simulink model "tractor_trailer_kinematics"  (R2024b)
settings: Solver=FixedStepAuto  StartTime=0.0  StopTime=10.0  FixedStep=0.01  RelTol=1e-3
values from neighbouring files (symbols this model uses):
  init_yaw = data.YawRad(1)    [initialize.m]
undefined symbols (not defined in the file or in its folder): param
settings Model: Creator=matve  LastModifiedBy=matve
settings RTWCC: GPUComputeCapability=3.5

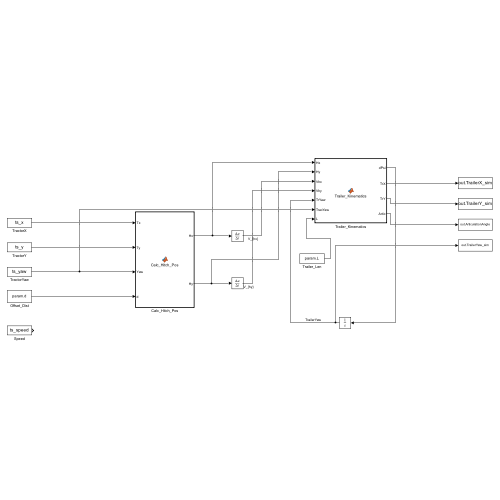
[thumbnail: Simulink's stored preview of the top-level diagram]
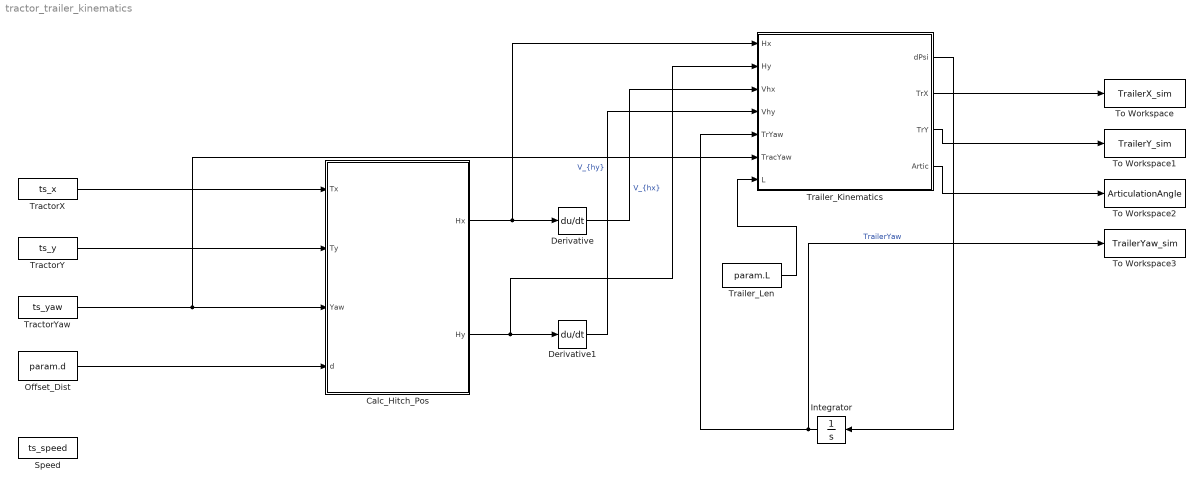
== system tractor_trailer_kinematics ==
  Calc_Hitch_Pos : MATLAB Function  TreatAsAtomicUnit=on
  Derivative : Derivative
  Derivative1 : Derivative
  Integrator : Integrator  InitialCondition=init_yaw
  Offset_Dist : Constant  Value=param.d
  Speed : FromWorkspace  VariableName=ts_speed  OutputAfterFinalValue=Holding final value
  To Workspace : ToWorkspace  VariableName=TrailerX_sim  SaveFormat=Timeseries  SampleTime=-1
  To Workspace1 : ToWorkspace  VariableName=TrailerY_sim  SaveFormat=Timeseries  SampleTime=-1
  To Workspace2 : ToWorkspace  VariableName=ArticulationAngle  SaveFormat=Timeseries  SampleTime=-1
  To Workspace3 : ToWorkspace  VariableName=TrailerYaw_sim  SaveFormat=Timeseries  SampleTime=-1
  TractorX : FromWorkspace  VariableName=ts_x
  TractorY : FromWorkspace  VariableName=ts_y
  TractorYaw : FromWorkspace  VariableName=ts_yaw
  Trailer_Kinematics : MATLAB Function  TreatAsAtomicUnit=on
  Trailer_Len : Constant  Value=param.L
  wires:
  TractorX/1 -> Calc_Hitch_Pos/1(Tx)
  TractorY/1 -> Calc_Hitch_Pos/2(Ty)
  TractorYaw/1 -> Trailer_Kinematics/6(TracYaw), Calc_Hitch_Pos/3(Yaw)
  Offset_Dist/1 -> Calc_Hitch_Pos/4(d)
  Calc_Hitch_Pos/1(Hx) -> Trailer_Kinematics/1(Hx), Derivative/1
  Calc_Hitch_Pos/2(Hy) -> Trailer_Kinematics/2(Hy), Derivative1/1
  Derivative/1 -> Trailer_Kinematics/3(Vhx)  "V_{hx}"
  Derivative1/1 -> Trailer_Kinematics/4(Vhy)  "V_{hy}"
  Integrator/1 -> To Workspace3/1, Trailer_Kinematics/5(TrYaw)  "TrailerYaw"
  Trailer_Len/1 -> Trailer_Kinematics/7(L)
  Trailer_Kinematics/1(dPsi) -> Integrator/1
  Trailer_Kinematics/2(TrX) -> To Workspace/1
  Trailer_Kinematics/3(TrY) -> To Workspace1/1
  Trailer_Kinematics/4(Artic) -> To Workspace2/1

== matlab function tractor_trailer_kinematics/Trailer_Kinematics ==
  data: Hx input; dPsi output; Hy input; Vhx input; Vhy input; TrYaw input; TracYaw input; L input; TrX output; TrY output; Artic output
function [dPsi, TrX, TrY, Artic] = Trailer_Kinematics(Hx, Hy, Vhx, Vhy, TrYaw, TracYaw, L)
    % 1. Calculate change in trailer angle (Yaw Rate)
    % Equation: dPsi = (1/L) * ( Vhy*cos(Psi) - Vhx*sin(Psi) )
    dPsi = (1/L) * (Vhy * cos(TrYaw) - Vhx * sin(TrYaw));

    % 2. Calculate Trailer Position
    TrX = Hx - L * cos(TrYaw);
    TrY = Hy - L * sin(TrYaw);

    % 3. Calculate Articulation Angle
    Artic = TracYaw - TrYaw;
end

== matlab function tractor_trailer_kinematics/Calc_Hitch_Pos ==
  data: Tx input; Hx output; Ty input; Yaw input; d input; Hy output
function [Hx, Hy] = Calc_Hitch_Pos(Tx, Ty, Yaw, d)
    % Calculates the global position of the 5th wheel (Hitch)
    % X_hitch = X_tractor - d * cos(theta)
    % Y_hitch = Y_tractor - d * sin(theta)

    Hx = Tx - d * cos(Yaw);
    Hy = Ty - d * sin(Yaw);
end
